simulink model "Vohmic"  (R2023a)
settings: Solver=VariableStepAuto  StartTime=0.0  StopTime=10.0  RelTol=1e-3
undefined symbols (not defined in the file): C
settings Model: Creator=meghn  LastModifiedBy=meghn

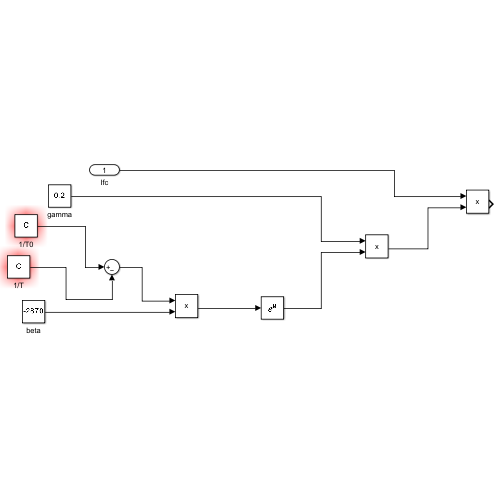
[thumbnail: Simulink's stored preview of the top-level diagram]
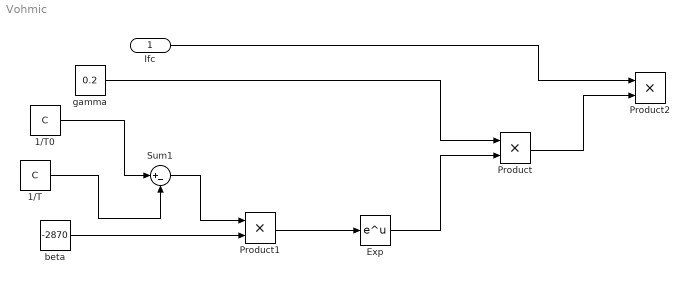
== system Vohmic ==
  Ifc : Inport
  1/T : Constant  Value=C
  1/T0 : Constant  Value=C
  Exp : Math
  Product : Product
  Product1 : Product
  Product2 : Product
  Sum1 : Sum  Inputs=|+-
  beta : Constant  Value=-2870
  gamma : Constant  Value=0.2
  wires:
  Ifc/1 -> Product2/1
  gamma/1 -> Product/1
  beta/1 -> Product1/2
  1/T0/1 -> Sum1/1
  1/T/1 -> Sum1/2
  Sum1/1 -> Product1/1
  Product1/1 -> Exp/1
  Exp/1 -> Product/2
  Product/1 -> Product2/2
